simulink model "untitled4"  (R2015a)
settings: Solver=ode45  StartTime=0.0  StopTime=1  RelTol=1e-3
libraries: powerlib x22
settings Model: Creator=MBK  LastModifiedBy=MBK
settings DataIOCC: LimitDataPoints=off

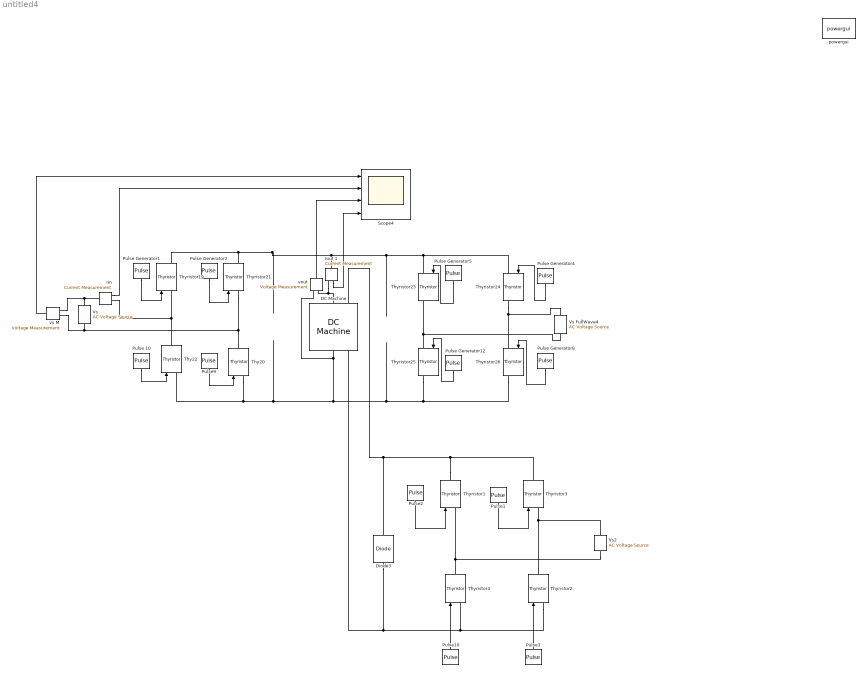
== system untitled4 ==
  "DC Machine " : powerlib/Machines/DC Machine  PresetModel=No  MechanicalLoad=Speed w  FieldType=Wound  ShowDetailedParameters=on  MeasurementBus=off  RLa="[ 0.6  0.120]"  RLf="[ 240  120]"  Laf=1.8  MachineConstant=Torque constant (N.m/A)  Ke=1.8  Kt=1.8  J=0.02215  Bm=0.002953  Tf=0.5161  w0=1  Ifinit=1  TsPowergui=0  TsBlock=-1
  Diode3 : powerlib/Power Electronics/Diode  Ron=0.001  Lon=0  Vf=0.8  IC=0  UseSnubber=off  Rs=500  Cs=250e-9  Measurements=off
  "Iin " : powerlib/Measurements/Current Measurement  PhasorSimulation=off  OutputType=Complex  PSBequivalent=0
  Iout 1 : powerlib/Measurements/Current Measurement  PhasorSimulation=off  OutputType=Complex  PSBequivalent=0
  Pulse 10 : DiscretePulseGenerator  PulseType=Time based  Amplitude=5  Period=0.02  PulseWidth=5  PhaseDelay=240*0.02/360
  Pulse Generator1 : DiscretePulseGenerator  PulseType=Time based  Amplitude=5  Period=0.02  PulseWidth=5  PhaseDelay=60*0.02/360
  Pulse Generator12 : DiscretePulseGenerator  PulseType=Time based  Amplitude=5  Period=0.02  PulseWidth=5  PhaseDelay=360*0.02/360
  Pulse Generator2 : DiscretePulseGenerator  PulseType=Time based  Amplitude=5  Period=0.02  PulseWidth=5  PhaseDelay=240*0.02/360
  Pulse Generator4 : DiscretePulseGenerator  PulseType=Time based  Amplitude=5  Period=0.02  PulseWidth=5  PhaseDelay=360*0.02/360
  Pulse Generator5 : DiscretePulseGenerator  PulseType=Time based  Amplitude=5  Period=0.02  PulseWidth=5  PhaseDelay=180*0.02/360
  Pulse Generator8 : DiscretePulseGenerator  PulseType=Time based  Amplitude=5  Period=0.02  PulseWidth=5  PhaseDelay=180*0.02/360
  Pulse1 : DiscretePulseGenerator  PulseType=Time based  Amplitude=5  Period=0.02  PulseWidth=5  PhaseDelay=240*0.02/360
  Pulse10 : DiscretePulseGenerator  PulseType=Time based  Amplitude=5  Period=0.02  PulseWidth=5  PhaseDelay=240*0.02/360
  Pulse2 : DiscretePulseGenerator  PulseType=Time based  Amplitude=5  Period=0.02  PulseWidth=5  PhaseDelay=60*0.02/360
  Pulse3 : DiscretePulseGenerator  PulseType=Time based  Amplitude=5  Period=0.02  PulseWidth=5  PhaseDelay=60*0.02/360
  Pulse9 : DiscretePulseGenerator  PulseType=Time based  Amplitude=5  Period=0.02  PulseWidth=5  PhaseDelay=60*0.02/360
  Scope4 : Scope  NumInputPorts=4
      settings: YMin=-400~-25~-50~-25  YMax=400~200~350~200  SaveName=ScopeData3
  Thy20 : powerlib/Power Electronics/Thyristor  Ron=0.001  Lon=0  Vf=0.8  IC=0  Rs=500  Cs=250e-9  Measurements=off
  Thy22 : powerlib/Power Electronics/Thyristor  Ron=0.001  Lon=0  Vf=0.8  IC=0  Rs=500  Cs=250e-9  Measurements=off
  Thyristor{1..4} (4 alike) : powerlib/Power Electronics/Thyristor  Ron=0.001  Lon=0  Vf=0.8  IC=0  Rs=500  Cs=250e-9  Measurements=off
  Thyristor{19,21,23..26} (6 alike) : powerlib/Power Electronics/Thyristor  Ron=0.001  Lon=0  Vf=0.8  IC=0  Rs=500  Cs=250e-9  Measurements=on
  "Vs " : powerlib/Electrical Sources/AC Voltage Source  Amplitude=220*sqrt(2)  Phase=0  Frequency=50  SampleTime=0  Measurements=None
  Vs FullWave4 : powerlib/Electrical Sources/AC Voltage Source  Amplitude=220*sqrt(2)  Phase=0  Frequency=50  SampleTime=0  Measurements=None
  Vs2 : powerlib/Electrical Sources/AC Voltage Source  Amplitude=220*sqrt(2)  Phase=0  Frequency=50  SampleTime=0  Measurements=None
  powergui : powerlib/powergui  Priority=1  SimulationMode=Continuous  SolverType=Tustin/Backward Euler (TBE)  SampleTime=50e-6  frequency=60  SPID=off  DisableSnubberDevices=off  DisableRonSwitches=off  DisableVfSwitches=off  SwTol=0  DisplayEquations=off  Interpol=off  methode=off  Ts=100  FunctionMessages=off  echomessages=off  HookPort=off  EnableUseOfTLC=off  x0status=blocks  frequencyindice=50  Pbase=100e6  ErrMax=1e-4  Iterations=50  UnitsV=kV  UnitsW=MW  buscounter=0  RestoreLinks=warning  ResistiveCurrentMeasurement=off  Frange=[0:2:500]  Ylog=off  Xlog=on  ShowGrid=off  save=off  variable=ZData  structure=0  ZoomFFT=off  StartTime=0.0  cycles=1  DisplayStyle=1  fundamental=60  FreqAxis=off  MaxFrequency=1000  frequencyindicesteady=1  RmsSteady=1  display=off
  "vout " : powerlib/Measurements/Voltage Measurement  PhasorSimulation=off  OutputType=Complex  PSBequivalent=0
  "vs M " : powerlib/Measurements/Voltage Measurement  PhasorSimulation=off  OutputType=Complex  PSBequivalent=0
  wires:
  Pulse9/1 -> Thy20/1
  "vs M "/1 -> Scope4/1
  "Iin "/1 -> Scope4/2
  "vout "/1 -> Scope4/3
  Iout 1/1 -> Scope4/4
  Pulse 10/1 -> Thy22/1
  Pulse Generator12/1 -> Thyristor25/1
  Pulse Generator1/1 -> Thyristor19/1
  Pulse Generator2/1 -> Thyristor21/1
  Pulse Generator4/1 -> Thyristor24/1
  Pulse Generator5/1 -> Thyristor23/1
  Pulse Generator8/1 -> Thyristor26/1
  Pulse3/1 -> Thyristor2/1
  Pulse10/1 -> Thyristor4/1
  Pulse1/1 -> Thyristor3/1
  Pulse2/1 -> Thyristor1/1
  connections:
  Thy22/RConn1 -- "Iin "/RConn1 -- Thyristor19/LConn1
  "Vs "/LConn1 -- Thyristor21/LConn1 -- Thy20/RConn1 -- "vs M "/LConn2
  "vout "/LConn2 -- "DC Machine "/RConn1 -- Thyristor25/RConn1 -- Thyristor26/RConn1 -- Thy22/LConn1 -- Thy20/LConn1
  "vs M "/LConn1 -- "Iin "/LConn1 -- "Vs "/RConn1
  Thyristor24/RConn1 -- Vs FullWave4/RConn1 -- Thyristor26/LConn1
  Vs FullWave4/LConn1 -- Thyristor23/RConn1 -- Thyristor25/LConn1
  Thyristor23/LConn1 -- Thyristor24/LConn1 -- Iout 1/LConn1 -- Thyristor19/RConn1 -- Thyristor21/RConn1
  Thyristor2/RConn1 -- Vs2/RConn1 -- Thyristor3/LConn1
  Thyristor4/RConn1 -- Thyristor1/LConn1 -- Vs2/LConn1
  Thyristor1/RConn1 -- Thyristor3/RConn1 -- "DC Machine "/LConn2 -- Diode3/RConn1
  Thyristor4/LConn1 -- Thyristor2/LConn1 -- "DC Machine "/RConn2 -- Diode3/LConn1
  "DC Machine "/LConn1 -- Iout 1/RConn1 -- "vout "/LConn1
